simulink model "PID_HW_EKF"  (R2024a)
settings: Solver=FixedStepAuto  StartTime=0.0  StopTime=inf  FixedStep=0.001  RelTol=1e-3  EnableMultiTasking=on
undefined symbols (not defined in the file): dev, Main, MAX_CONTROL_ANGLE_RATE_ROLL, P, pwm_output0, R_p_x, Saturation_I_RP_Max, Saturation_I_RP_Min
libraries: slpidlib x5, px4Sensorslib x2, px4lib x1
settings Model: SimulationMode=external  ExtModeTrigDuration=10  Creator=ArriGE66  LastModifiedBy=sebas
settings SolverCC: PositivePriorityOrder=on
settings OptimizationCC: EnhancedBackFolding=on  PassReuseOutputArgsAs=Individual arguments  ZeroExternalMemoryAtStartup=off  ZeroInternalMemoryAtStartup=off  MaxStackSize=64  OptimizeBlockOrder=speed  DifferentSizesBufferReuse=on  EfficientTunableParamExpr=on
settings DebuggingCC: ParameterTunabilityLossMsg=error
settings HardwareCC: ProdBitPerPointer=32  ProdBitPerSizeT=32  ProdBitPerPtrDiffT=32  ProdLargestAtomicInteger=Long  ProdLargestAtomicFloat=Double  ProdWordSize=32  ProdLongLongMode=on  ProdHWDeviceType=ARM Compatible->ARM Cortex
settings SFSimCC: MATLABDynamicMemAlloc=off  SimTargetLang=C++
settings RTWCC: Description=Embedded Coder  SystemTargetFile=ert.tlc  HardwareBoard=PX4 Cube Orange  TemplateMakefile=ert_default_tmf  Toolchain=GNU Tools for PX4 Autopilots  TargetLang=C++  GPUComputeCapability=3.5
settings CodeAppCC: ForceParamTrailComments=on  IgnoreCustomStorageClasses=off  OperatorAnnotations=on  SimulinkDataObjDesc=on  SFDataObjDesc=on  InsertBlockDesc=on
settings ERTTargetCC: ExtMode=on  ExtModeTransport=3  ExtModeStaticAlloc=on  ExtModeStaticAllocSize=1024  ExtModeMexFile=ext_xcp  ExtModeMexArgs=1 COM10 3000000  ExtModeIntrfLevel=Level2 - Open

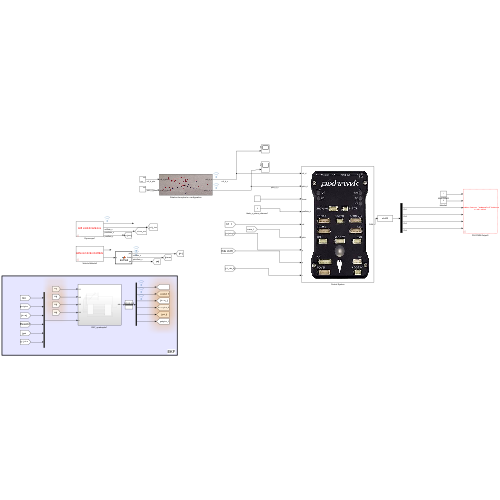
[thumbnail: Simulink's stored preview of the top-level diagram]
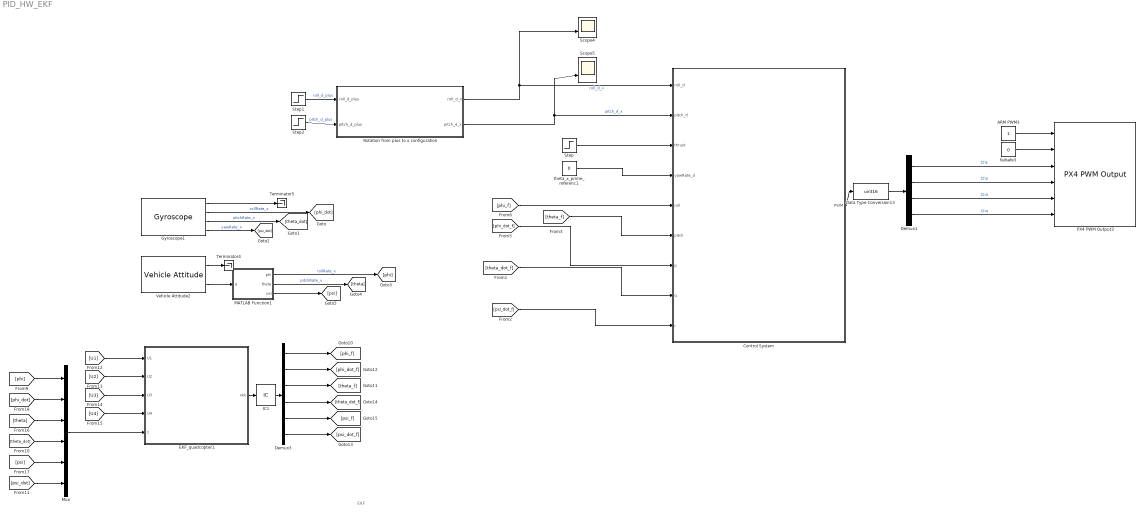
== system PID_HW_EKF ==
  note: EKF
  ARM PWM3 : Constant  OutDataTypeStr=boolean  SampleTime=0.002
  Control System : Subsystem
      mask Display: image('icon\pixhawk.png');
  Data Type Conversion13 : DataTypeConversion  OutDataTypeStr=uint16  SaturateOnIntegerOverflow=off  RndMeth=Floor
  Demux1 : Demux
  Demux3 : Demux  Outputs=6
  EKF_quadcopter1 : Subsystem
  Gyroscope1 : px4Sensorslib/Gyroscope  uorbTimeStamp=off  BlockingMode=off  BlockTimeout=1e-3  sampleTime=0.002
  IC1 : InitialCondition  Value=[0;0;0;0;0;0]
  MATLAB Function1 : MATLAB Function  TreatAsAtomicUnit=on
  Mux : Mux  Inputs=6
  PX4 PWM Output3 : px4lib/PX4 PWM Output  pwmDevice=Main (/dev/pwm_output0)  pwmChannel1_=on  pwmChannel2_=on  pwmChannel3_=on  pwmChannel4_=on  pwmChannel5_=off  pwmChannel6_=off  pwmChannel7_=off  pwmChannel8_=off  forceTerminateFailsafe=off  outputErrorStatus=off
  Rotation from plus to x configuration : Subsystem
      mask Display: image('rotation_matrix.jpg');
  Scope4 : Scope  NumInputPorts=2
  Scope5 : Scope  NumInputPorts=2
  Step : Step  After=0.6085  SampleTime=0.002
  Step1 : Step  Time=0  After=0  SampleTime=0.002
  Step2 : Step  Time=2  After=0  SampleTime=0.002
  Terminator4 : Terminator
  Terminator5 : Terminator
  Vehicle Attitude2 : px4Sensorslib/Vehicle Attitude  rollRate=off  pitchRate=off  yawRate=off  quaternion=on  uorbTimeStamp=off  BlockingMode=off  BlockTimeout=0.001  sampleTime=0.002
  failsafe3 : Constant  Value=0  OutDataTypeStr=boolean  SampleTime=0.002
  theta_x_prime_referenc1 : Constant  Value=0  SampleTime=0.002
  wires:
  Control System/1(PWM) -> Data Type Conversion13/1
  Data Type Conversion13/1 -> Demux1/1
  Demux1/1 -> PX4 PWM Output3/3  "Ch1"
  Demux1/2 -> PX4 PWM Output3/4  "Ch2"
  ARM PWM3/1 -> PX4 PWM Output3/1
  failsafe3/1 -> PX4 PWM Output3/2
  Step/1 -> Control System/3(thrust)
  theta_x_prime_referenc1/1 -> Control System/4(yawRate_d)
  Demux1/3 -> PX4 PWM Output3/5  "Ch3"
  Demux1/4 -> PX4 PWM Output3/6  "Ch4"
  Rotation from plus to x configuration/2(pitch_d_x) -> Control System/2(pitch_d), Scope5/2  "pitch_d_x"
  Rotation from plus to x configuration/1(roll_d_x) -> Control System/1(roll_d), Scope4/2  "roll_d_x"
  Step1/1 -> Rotation from plus to x configuration/1(roll_d_plus)  "roll_d_plus"
  Step2/1 -> Rotation from plus to x configuration/2(pitch_d_plus)  "pitch_d_plus"
  MATLAB Function1/2(theta) -> [theta]  "pitchRate_x"
  MATLAB Function1/1(phi) -> [phi]  "rollRate_x"
  Gyroscope1/1 -> Terminator5/1
  Vehicle Attitude2/2 -> MATLAB Function1/1(q)
  Vehicle Attitude2/1 -> Terminator4/1
  Gyroscope1/3 -> [theta_dot]  "pitchRate_x"
  Gyroscope1/2 -> [phi_dot]  "rollRate_x"
  Gyroscope1/4 -> [psi_dot]  "yawRate_x"
  MATLAB Function1/3(psi) -> [psi]
  [U1] -> EKF_quadcopter1/1(U1)
  Mux/1 -> EKF_quadcopter1/5(z)
  [phi] -> Mux/1
  [U3] -> EKF_quadcopter1/3(U3)
  [psi_dot] -> Mux/6
  [U2] -> EKF_quadcopter1/2(U2)
  [psi] -> Mux/5
  Demux3/5 -> [psi_f]
  [theta] -> Mux/3
  [theta_dot] -> Mux/4
  Demux3/2 -> [phi_dot_f]
  Demux3/1 -> [phi_f]
  Demux3/6 -> [psi_dot_f]
  EKF_quadcopter1/1(xkk) -> IC1/1
  Demux3/3 -> [theta_f]
  [phi_dot] -> Mux/2
  Demux3/4 -> [theta_dot_f]
  IC1/1 -> Demux3/1
  [U4] -> EKF_quadcopter1/4(U4)
  [theta_dot_f] -> Control System/8(q)
  [theta_f] -> Control System/6(pitch)
  [psi_dot_f] -> Control System/9(r)
  [phi_f] -> Control System/5(roll)
  [phi_dot_f] -> Control System/7(p)

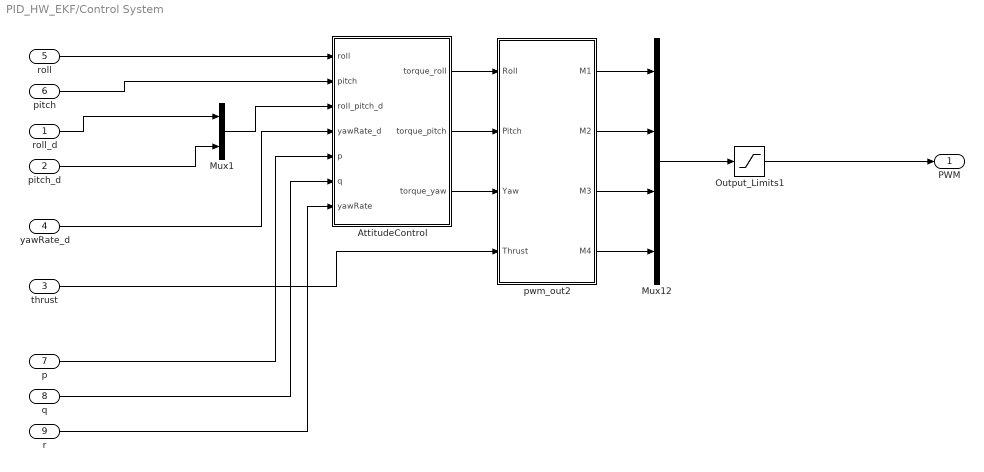
== system PID_HW_EKF/Control System ==
  roll_d : Inport  PortDimensions=1
  pitch_d : Inport  Port=2  PortDimensions=1
  thrust : Inport  Port=3  PortDimensions=1
  yawRate_d : Inport  Port=4  PortDimensions=1
  roll : Inport  Port=5  PortDimensions=1
  pitch : Inport  Port=6  PortDimensions=1
  p : Inport  Port=7  PortDimensions=1
  q : Inport  Port=8  PortDimensions=1
  r : Inport  Port=9  PortDimensions=1
  AttitudeControl : Subsystem
  Mux1 : Mux  Inputs=2
  Mux12 : Mux
  Output_Limits1 : Saturate  UpperLimit=2000  LowerLimit=1000  LinearizeAsGain=off
  pwm_out2 : MATLAB Function  SystemSampleTime=0.004
  PWM : Outport  VectorParamsAs1DForOutWhenUnconnected=off
  wires:
  thrust/1 -> pwm_out2/4(Thrust)
  Mux12/1 -> Output_Limits1/1
  AttitudeControl/2(torque_pitch) -> pwm_out2/2(Pitch)
  AttitudeControl/1(torque_roll) -> pwm_out2/1(Roll)
  pwm_out2/1(M1) -> Mux12/1
  pwm_out2/3(M3) -> Mux12/3
  pwm_out2/2(M2) -> Mux12/2
  r/1 -> AttitudeControl/7(yawRate)
  AttitudeControl/3(torque_yaw) -> pwm_out2/3(Yaw)
  Mux1/1 -> AttitudeControl/3(roll_pitch_d)
  q/1 -> AttitudeControl/6(q)
  yawRate_d/1 -> AttitudeControl/4(yawRate_d)
  p/1 -> AttitudeControl/5(p)
  pwm_out2/4(M4) -> Mux12/4
  pitch/1 -> AttitudeControl/2(pitch)
  roll/1 -> AttitudeControl/1(roll)
  Output_Limits1/1 -> PWM/1
  roll_d/1 -> Mux1/1
  pitch_d/1 -> Mux1/2

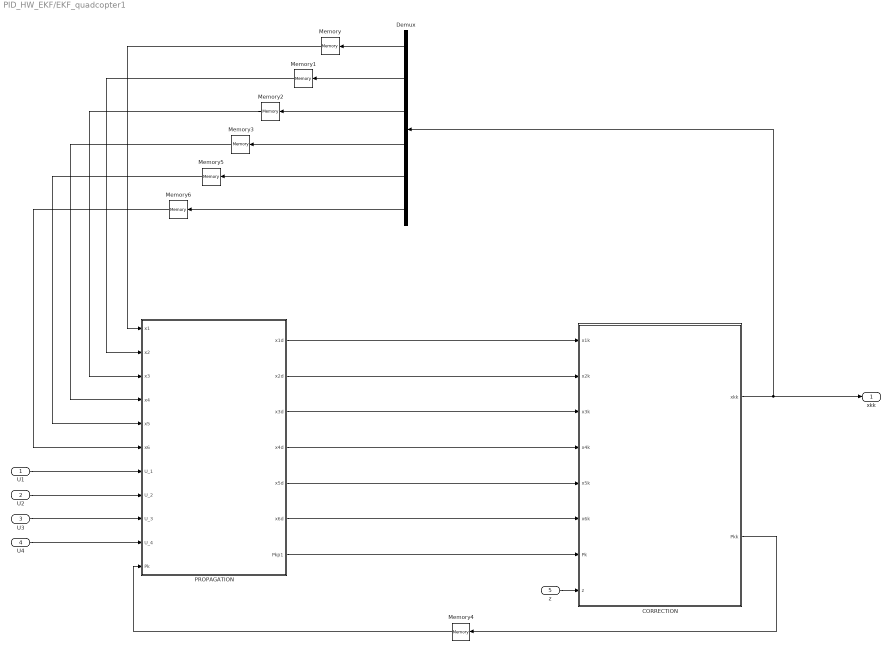
== system PID_HW_EKF/EKF_quadcopter1 ==
  U1 : Inport
  U2 : Inport  Port=2
  U3 : Inport  Port=3
  U4 : Inport  Port=4
  z : Inport  Port=5
  CORRECTION : MATLAB Function  TreatAsAtomicUnit=on
  Demux : Demux  Outputs=6
  Memory{,1..3,5..6} (6 alike) : Memory
  Memory4 : Memory  InitialCondition=P
  PROPAGATION : MATLAB Function  TreatAsAtomicUnit=on
  xkk : Outport
  wires:
  PROPAGATION/1(x1d) -> CORRECTION/1(x1k)
  PROPAGATION/2(x2d) -> CORRECTION/2(x2k)
  PROPAGATION/3(x3d) -> CORRECTION/3(x3k)
  PROPAGATION/4(x4d) -> CORRECTION/4(x4k)
  Memory4/1 -> PROPAGATION/11(Pk)
  U1/1 -> PROPAGATION/7(U_1)
  U2/1 -> PROPAGATION/8(U_2)
  U3/1 -> PROPAGATION/9(U_3)
  U4/1 -> PROPAGATION/10(U_4)
  PROPAGATION/7(Pkp1) -> CORRECTION/7(Pk)
  CORRECTION/2(Pkk) -> Memory4/1
  z/1 -> CORRECTION/8(z)
  Demux/1 -> Memory/1
  Demux/2 -> Memory1/1
  Demux/3 -> Memory2/1
  Demux/4 -> Memory3/1
  CORRECTION/1(xkk) -> Demux/1, xkk/1
  Memory/1 -> PROPAGATION/1(x1)
  Memory1/1 -> PROPAGATION/2(x2)
  Memory2/1 -> PROPAGATION/3(x3)
  Memory3/1 -> PROPAGATION/4(x4)
  PROPAGATION/6(x6d) -> CORRECTION/6(x6k)
  PROPAGATION/5(x5d) -> CORRECTION/5(x5k)
  Demux/5 -> Memory5/1
  Memory5/1 -> PROPAGATION/5(x5)
  Demux/6 -> Memory6/1
  Memory6/1 -> PROPAGATION/6(x6)

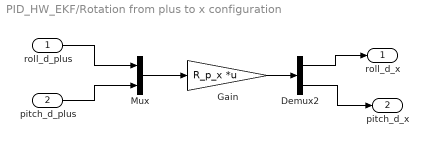
== system PID_HW_EKF/Rotation from plus to x configuration ==
  roll_d_plus : Inport
  pitch_d_plus : Inport  Port=2
  Demux2 : Demux  Outputs=2
  Gain : Gain  Gain=R_p_x  Multiplication=Matrix(K*u) (u vector)
  Mux : Mux  Inputs=2
  roll_d_x : Outport
  pitch_d_x : Outport  Port=2
  wires:
  roll_d_plus/1 -> Mux/1
  Mux/1 -> Gain/1
  Demux2/1 -> roll_d_x/1
  Gain/1 -> Demux2/1
  pitch_d_plus/1 -> Mux/2
  Demux2/2 -> pitch_d_x/1

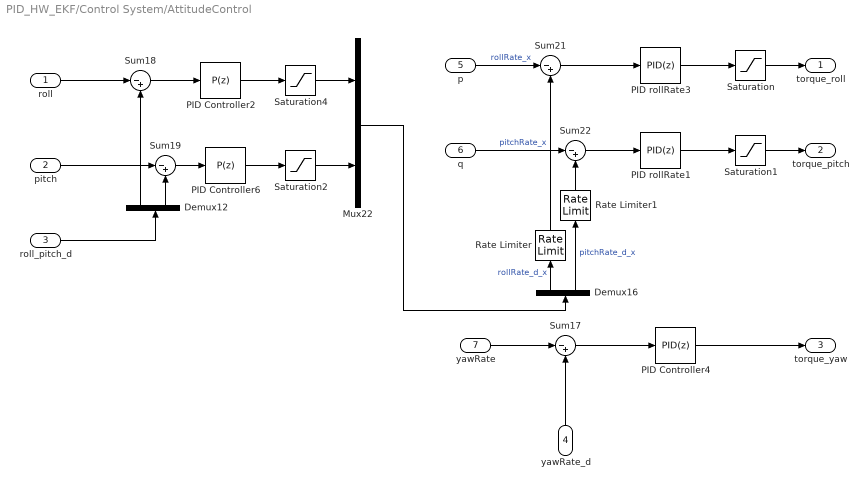
== system PID_HW_EKF/Control System/AttitudeControl ==
  roll : Inport
  pitch : Inport  Port=2
  roll_pitch_d : Inport  Port=3
  yawRate_d : Inport  Port=4
  p : Inport  Port=5
  q : Inport  Port=6
  yawRate : Inport  Port=7
  Demux12 : Demux  Outputs=2
  Demux16 : Demux  Outputs=2
  Mux22 : Mux  Inputs=2
  PID Controller2 : slpidlib/PID Controller  Controller=P  Form=Parallel  TimeDomain=Discrete-time  UseExternalTs=off  SampleTime=-1  IntegratorMethod=Forward Euler  FilterMethod=Forward Euler  ControllerParametersSource=internal  P=2.809480033162003  I=1  UseKiTs=off  D=0  UseExternalDerivativeSource=off  N=100  UseFilter=on  TunerSelectOption=Transfer Function Based (PID Tuner App)  InitialConditionSource=internal  InitialConditionForIntegrator=0  InitialConditionForFilter=0  DifferentiatorICPrevScaledInput=0  ExternalReset=none  TrackingMode=off  Kt=1  LimitOutput=off  SatLimitsSource=internal  UpperSaturationLimit=inf  LowerSaturationLimit=-inf  LinearizeAsGain=on  AntiWindupMode=none  Kb=1  LimitIntegrator=off  UpperIntegratorSaturationLimit=inf  LowerIntegratorSaturationLimit=-inf  POutMin=[]  POutMax=[]  IOutMin=[]  IOutMax=[]  DOutMin=[]  DOutMax=[]  NOutMin=[]  NOutMax=[]  SumOutMin=[]  SumOutMax=[]  SaturationOutMin=[]  SaturationOutMax=[]  PParamMin=[]  PParamMax=[]  IParamMin=[]  IParamMax=[]  DParamMin=[]  DParamMax=[]  NParamMin=[]  NParamMax=[]  KbParamMin=[]  KbParamMax=[]  KtParamMin=[]  KtParamMax=[]  KbOutMin=[]  KbOutMax=[]  KtOutMin=[]  KtOutMax=[]  IntegratorOutMin=[]  IntegratorOutMax=[]  FilterOutMin=[]  FilterOutMax=[]  SumI1OutMin=[]  SumI1OutMax=[]  SumI2OutMin=[]  SumI2OutMax=[]  SumI3OutMin=[]  SumI3OutMax=[]  SumI4OutMin=[]  SumI4OutMax=[]  SumDOutMin=[]  SumDOutMax=[]  DifferentiatorOutMin=[]  DifferentiatorOutMax=[]  FilterDiffOutCoefMin=[]  FilterDiffOutCoefMax=[]  ReciprocalOutMin=[]  ReciprocalOutMax=[]  SumDenOutMin=[]  SumDenOutMax=[]  SumNumOutMin=[]  SumNumOutMax=[]  DivideOutMin=[]  DivideOutMax=[]  UdiffTsProdOutMin=[]  UdiffTsProdOutMax=[]  NTsProdOutMin=[]  NTsProdOutMax=[]  UintegralTsProdOutMin=[]  UintegralTsProdOutMax=[]  UngainTsProdOutMin=[]  UngainTsProdOutMax=[]  ClampingZeroOutDataTypeStr=Inherit: Inherit via back propagation  ClampingZeroOutMin=[]  ClampingZeroOutMax=[]  FilterDenConstantOutDataTypeStr=Inherit: Inherit via back propagation  FilterDenConstantOutMin=[]  FilterDenConstantOutMax=[]  PCopyOutDataTypeStr=Inherit: Inherit via back propagation  PCopyOutMin=[]  PCopyOutMax=[]  NCopyOutDataTypeStr=Inherit: Inherit via back propagation  NCopyOutMin=[]  NCopyOutMax=[]  IntegratorContinuousStateAttributes=''  IntegratorStateMustResolveToSignalObject=off  IntegratorRTWStateStorageClass=Auto  FilterContinuousStateAttributes=''  FilterStateMustResolveToSignalObject=off  FilterRTWStateStorageClass=Auto  ParallelPVariant=InternalParameters  IdealPVariant=Disabled  IVariant=Disabled  DVariant=Disabled  IntegratorVariant=Disabled  SatVariant=Disabled  AWVariant=Disabled  PCopyVariant=Disabled  TRVariant=Disabled  FdbkBlocksVariant=Forward  IdealPFdbkVariant=Disabled  SatFdbkVariant=Disabled  DerivativeFilterVariant=Disabled  NVariant=Disabled  NCopyVariant=Disabled_SignalSpec  FilterICVariant=Disabled  IntegratorICVariant=Disabled  ExternalResetVariant=Disabled  TRSumVariant=Passthrough  SumFdbkVariant=Disabled  SumVariant=Passthrough_P  TsampFilterVariant=InternalTs  TsampNgainVariant=Passthrough  TsampIntegralVariant=Disabled_SignalSpec  ExternalSaturationOutDataTypeStr=Inherit: Same as second input  DerivativeSourceVariant=Disabled
  PID Controller4 : slpidlib/PID Controller  Controller=PID  Form=Parallel  TimeDomain=Discrete-time  UseExternalTs=off  SampleTime=-1  IntegratorMethod=Forward Euler  FilterMethod=Forward Euler  ControllerParametersSource=internal  P=7.29164976020127  I=128.977906817925  UseKiTs=off  D=0.0102787963324955  UseExternalDerivativeSource=off  N=308.658502253511  UseFilter=on  TunerSelectOption=Transfer Function Based (PID Tuner App)  InitialConditionSource=internal  InitialConditionForIntegrator=0  InitialConditionForFilter=0  DifferentiatorICPrevScaledInput=0  ExternalReset=none  TrackingMode=off  Kt=1  LimitOutput=off  SatLimitsSource=internal  UpperSaturationLimit=Saturation_I_RP_Max  LowerSaturationLimit=Saturation_I_RP_Min  LinearizeAsGain=on  AntiWindupMode=none  Kb=1  LimitIntegrator=off  UpperIntegratorSaturationLimit=inf  LowerIntegratorSaturationLimit=-inf  POutMin=[]  POutMax=[]  IOutMin=[]  IOutMax=[]  DOutMin=[]  DOutMax=[]  NOutMin=[]  NOutMax=[]  SumOutMin=[]  SumOutMax=[]  SaturationOutMin=[]  SaturationOutMax=[]  PParamMin=[]  PParamMax=[]  IParamMin=[]  IParamMax=[]  DParamMin=[]  DParamMax=[]  NParamMin=[]  NParamMax=[]  KbParamMin=[]  KbParamMax=[]  KtParamMin=[]  KtParamMax=[]  KbOutMin=[]  KbOutMax=[]  KtOutMin=[]  KtOutMax=[]  IntegratorOutMin=[]  IntegratorOutMax=[]  FilterOutMin=[]  FilterOutMax=[]  SumI1OutMin=[]  SumI1OutMax=[]  SumI2OutMin=[]  SumI2OutMax=[]  SumI3OutMin=[]  SumI3OutMax=[]  SumI4OutMin=[]  SumI4OutMax=[]  SumDOutMin=[]  SumDOutMax=[]  DifferentiatorOutMin=[]  DifferentiatorOutMax=[]  FilterDiffOutCoefMin=[]  FilterDiffOutCoefMax=[]  ReciprocalOutMin=[]  ReciprocalOutMax=[]  SumDenOutMin=[]  SumDenOutMax=[]  SumNumOutMin=[]  SumNumOutMax=[]  DivideOutMin=[]  DivideOutMax=[]  UdiffTsProdOutMin=[]  UdiffTsProdOutMax=[]  NTsProdOutMin=[]  NTsProdOutMax=[]  UintegralTsProdOutMin=[]  UintegralTsProdOutMax=[]  UngainTsProdOutMin=[]  UngainTsProdOutMax=[]  ClampingZeroOutDataTypeStr=Inherit: Inherit via back propagation  ClampingZeroOutMin=[]  ClampingZeroOutMax=[]  FilterDenConstantOutDataTypeStr=Inherit: Inherit via back propagation  FilterDenConstantOutMin=[]  FilterDenConstantOutMax=[]  PCopyOutDataTypeStr=Inherit: Inherit via back propagation  PCopyOutMin=[]  PCopyOutMax=[]  NCopyOutDataTypeStr=Inherit: Inherit via back propagation  NCopyOutMin=[]  NCopyOutMax=[]  IntegratorContinuousStateAttributes=''  IntegratorStateMustResolveToSignalObject=off  IntegratorRTWStateStorageClass=Auto  FilterContinuousStateAttributes=''  FilterStateMustResolveToSignalObject=off  FilterRTWStateStorageClass=Auto  ParallelPVariant=InternalParameters  IdealPVariant=Disabled  IVariant=InternalParameters  DVariant=InternalParameters  IntegratorVariant=Discrete  SatVariant=Disabled  AWVariant=Passthrough  PCopyVariant=Disabled  TRVariant=Disabled  FdbkBlocksVariant=Forward  IdealPFdbkVariant=Disabled  SatFdbkVariant=Disabled  DerivativeFilterVariant=ForwardEulerFilter  NVariant=InternalParameters  NCopyVariant=Disabled  FilterICVariant=InternalICsFilter  IntegratorICVariant=InternalICs  ExternalResetVariant=Disabled  TRSumVariant=Passthrough  SumFdbkVariant=Disabled  SumVariant=Sum_PID  TsampFilterVariant=InternalTs  TsampNgainVariant=Passthrough  TsampIntegralVariant=Disabled_SignalSpec  ExternalSaturationOutDataTypeStr=Inherit: Same as second input  DerivativeSourceVariant=ErrorSignal
  PID Controller6 : slpidlib/PID Controller  Controller=P  Form=Parallel  TimeDomain=Discrete-time  UseExternalTs=off  SampleTime=-1  IntegratorMethod=Forward Euler  FilterMethod=Forward Euler  ControllerParametersSource=internal  P=2.809480033162003  I=1  UseKiTs=off  D=0  UseExternalDerivativeSource=off  N=100  UseFilter=on  TunerSelectOption=Transfer Function Based (PID Tuner App)  InitialConditionSource=internal  InitialConditionForIntegrator=0  InitialConditionForFilter=0  DifferentiatorICPrevScaledInput=0  ExternalReset=none  TrackingMode=off  Kt=1  LimitOutput=off  SatLimitsSource=internal  UpperSaturationLimit=inf  LowerSaturationLimit=-inf  LinearizeAsGain=on  AntiWindupMode=none  Kb=1  LimitIntegrator=off  UpperIntegratorSaturationLimit=inf  LowerIntegratorSaturationLimit=-inf  POutMin=[]  POutMax=[]  IOutMin=[]  IOutMax=[]  DOutMin=[]  DOutMax=[]  NOutMin=[]  NOutMax=[]  SumOutMin=[]  SumOutMax=[]  SaturationOutMin=[]  SaturationOutMax=[]  PParamMin=[]  PParamMax=[]  IParamMin=[]  IParamMax=[]  DParamMin=[]  DParamMax=[]  NParamMin=[]  NParamMax=[]  KbParamMin=[]  KbParamMax=[]  KtParamMin=[]  KtParamMax=[]  KbOutMin=[]  KbOutMax=[]  KtOutMin=[]  KtOutMax=[]  IntegratorOutMin=[]  IntegratorOutMax=[]  FilterOutMin=[]  FilterOutMax=[]  SumI1OutMin=[]  SumI1OutMax=[]  SumI2OutMin=[]  SumI2OutMax=[]  SumI3OutMin=[]  SumI3OutMax=[]  SumI4OutMin=[]  SumI4OutMax=[]  SumDOutMin=[]  SumDOutMax=[]  DifferentiatorOutMin=[]  DifferentiatorOutMax=[]  FilterDiffOutCoefMin=[]  FilterDiffOutCoefMax=[]  ReciprocalOutMin=[]  ReciprocalOutMax=[]  SumDenOutMin=[]  SumDenOutMax=[]  SumNumOutMin=[]  SumNumOutMax=[]  DivideOutMin=[]  DivideOutMax=[]  UdiffTsProdOutMin=[]  UdiffTsProdOutMax=[]  NTsProdOutMin=[]  NTsProdOutMax=[]  UintegralTsProdOutMin=[]  UintegralTsProdOutMax=[]  UngainTsProdOutMin=[]  UngainTsProdOutMax=[]  ClampingZeroOutDataTypeStr=Inherit: Inherit via back propagation  ClampingZeroOutMin=[]  ClampingZeroOutMax=[]  FilterDenConstantOutDataTypeStr=Inherit: Inherit via back propagation  FilterDenConstantOutMin=[]  FilterDenConstantOutMax=[]  PCopyOutDataTypeStr=Inherit: Inherit via back propagation  PCopyOutMin=[]  PCopyOutMax=[]  NCopyOutDataTypeStr=Inherit: Inherit via back propagation  NCopyOutMin=[]  NCopyOutMax=[]  IntegratorContinuousStateAttributes=''  IntegratorStateMustResolveToSignalObject=off  IntegratorRTWStateStorageClass=Auto  FilterContinuousStateAttributes=''  FilterStateMustResolveToSignalObject=off  FilterRTWStateStorageClass=Auto  ParallelPVariant=InternalParameters  IdealPVariant=Disabled  IVariant=Disabled  DVariant=Disabled  IntegratorVariant=Disabled  SatVariant=Disabled  AWVariant=Disabled  PCopyVariant=Disabled  TRVariant=Disabled  FdbkBlocksVariant=Forward  IdealPFdbkVariant=Disabled  SatFdbkVariant=Disabled  DerivativeFilterVariant=Disabled  NVariant=Disabled  NCopyVariant=Disabled_SignalSpec  FilterICVariant=Disabled  IntegratorICVariant=Disabled  ExternalResetVariant=Disabled  TRSumVariant=Passthrough  SumFdbkVariant=Disabled  SumVariant=Passthrough_P  TsampFilterVariant=InternalTs  TsampNgainVariant=Passthrough  TsampIntegralVariant=Disabled_SignalSpec  ExternalSaturationOutDataTypeStr=Inherit: Same as second input  DerivativeSourceVariant=Disabled
  PID rollRate1 : slpidlib/PID Controller  Controller=PID  Form=Parallel  TimeDomain=Discrete-time  UseExternalTs=off  SampleTime=-1  IntegratorMethod=Forward Euler  FilterMethod=Forward Euler  ControllerParametersSource=internal  P=7.82928757295584  I=30.614354689847  UseKiTs=off  D=-0.0391699970557117  UseExternalDerivativeSource=off  N=24.5460626191563  UseFilter=on  TunerSelectOption=Transfer Function Based (PID Tuner App)  InitialConditionSource=internal  InitialConditionForIntegrator=0  InitialConditionForFilter=0  DifferentiatorICPrevScaledInput=0  ExternalReset=none  TrackingMode=off  Kt=1  LimitOutput=off  SatLimitsSource=internal  UpperSaturationLimit=Saturation_I_RP_Max  LowerSaturationLimit=Saturation_I_RP_Min  LinearizeAsGain=on  AntiWindupMode=none  Kb=1  LimitIntegrator=off  UpperIntegratorSaturationLimit=inf  LowerIntegratorSaturationLimit=-inf  POutMin=[]  POutMax=[]  IOutMin=[]  IOutMax=[]  DOutMin=[]  DOutMax=[]  NOutMin=[]  NOutMax=[]  SumOutMin=[]  SumOutMax=[]  SaturationOutMin=[]  SaturationOutMax=[]  PParamMin=[]  PParamMax=[]  IParamMin=[]  IParamMax=[]  DParamMin=[]  DParamMax=[]  NParamMin=[]  NParamMax=[]  KbParamMin=[]  KbParamMax=[]  KtParamMin=[]  KtParamMax=[]  KbOutMin=[]  KbOutMax=[]  KtOutMin=[]  KtOutMax=[]  IntegratorOutMin=[]  IntegratorOutMax=[]  FilterOutMin=[]  FilterOutMax=[]  SumI1OutMin=[]  SumI1OutMax=[]  SumI2OutMin=[]  SumI2OutMax=[]  SumI3OutMin=[]  SumI3OutMax=[]  SumI4OutMin=[]  SumI4OutMax=[]  SumDOutMin=[]  SumDOutMax=[]  DifferentiatorOutMin=[]  DifferentiatorOutMax=[]  FilterDiffOutCoefMin=[]  FilterDiffOutCoefMax=[]  ReciprocalOutMin=[]  ReciprocalOutMax=[]  SumDenOutMin=[]  SumDenOutMax=[]  SumNumOutMin=[]  SumNumOutMax=[]  DivideOutMin=[]  DivideOutMax=[]  UdiffTsProdOutMin=[]  UdiffTsProdOutMax=[]  NTsProdOutMin=[]  NTsProdOutMax=[]  UintegralTsProdOutMin=[]  UintegralTsProdOutMax=[]  UngainTsProdOutMin=[]  UngainTsProdOutMax=[]  ClampingZeroOutDataTypeStr=Inherit: Inherit via back propagation  ClampingZeroOutMin=[]  ClampingZeroOutMax=[]  FilterDenConstantOutDataTypeStr=Inherit: Inherit via back propagation  FilterDenConstantOutMin=[]  FilterDenConstantOutMax=[]  PCopyOutDataTypeStr=Inherit: Inherit via back propagation  PCopyOutMin=[]  PCopyOutMax=[]  NCopyOutDataTypeStr=Inherit: Inherit via back propagation  NCopyOutMin=[]  NCopyOutMax=[]  IntegratorContinuousStateAttributes=''  IntegratorStateMustResolveToSignalObject=off  IntegratorRTWStateStorageClass=Auto  FilterContinuousStateAttributes=''  FilterStateMustResolveToSignalObject=off  FilterRTWStateStorageClass=Auto  ParallelPVariant=InternalParameters  IdealPVariant=Disabled  IVariant=InternalParameters  DVariant=InternalParameters  IntegratorVariant=Discrete  SatVariant=Disabled  AWVariant=Passthrough  PCopyVariant=Disabled  TRVariant=Disabled  FdbkBlocksVariant=Forward  IdealPFdbkVariant=Disabled  SatFdbkVariant=Disabled  DerivativeFilterVariant=ForwardEulerFilter  NVariant=InternalParameters  NCopyVariant=Disabled  FilterICVariant=InternalICsFilter  IntegratorICVariant=InternalICs  ExternalResetVariant=Disabled  TRSumVariant=Passthrough  SumFdbkVariant=Disabled  SumVariant=Sum_PID  TsampFilterVariant=InternalTs  TsampNgainVariant=Passthrough  TsampIntegralVariant=Disabled_SignalSpec  ExternalSaturationOutDataTypeStr=Inherit: Same as second input  DerivativeSourceVariant=ErrorSignal
  PID rollRate3 : slpidlib/PID Controller  Controller=PID  Form=Parallel  TimeDomain=Discrete-time  UseExternalTs=off  SampleTime=-1  IntegratorMethod=Forward Euler  FilterMethod=Forward Euler  ControllerParametersSource=internal  P=7.82928757295584  I=30.614354689847  UseKiTs=off  D=-0.0391699970557117  UseExternalDerivativeSource=off  N=24.5460626191563  UseFilter=on  TunerSelectOption=Transfer Function Based (PID Tuner App)  InitialConditionSource=internal  InitialConditionForIntegrator=0  InitialConditionForFilter=0  DifferentiatorICPrevScaledInput=0  ExternalReset=none  TrackingMode=off  Kt=1  LimitOutput=off  SatLimitsSource=internal  UpperSaturationLimit=Saturation_I_RP_Max  LowerSaturationLimit=Saturation_I_RP_Min  LinearizeAsGain=on  AntiWindupMode=none  Kb=1  LimitIntegrator=off  UpperIntegratorSaturationLimit=inf  LowerIntegratorSaturationLimit=-inf  POutMin=[]  POutMax=[]  IOutMin=[]  IOutMax=[]  DOutMin=[]  DOutMax=[]  NOutMin=[]  NOutMax=[]  SumOutMin=[]  SumOutMax=[]  SaturationOutMin=[]  SaturationOutMax=[]  PParamMin=[]  PParamMax=[]  IParamMin=[]  IParamMax=[]  DParamMin=[]  DParamMax=[]  NParamMin=[]  NParamMax=[]  KbParamMin=[]  KbParamMax=[]  KtParamMin=[]  KtParamMax=[]  KbOutMin=[]  KbOutMax=[]  KtOutMin=[]  KtOutMax=[]  IntegratorOutMin=[]  IntegratorOutMax=[]  FilterOutMin=[]  FilterOutMax=[]  SumI1OutMin=[]  SumI1OutMax=[]  SumI2OutMin=[]  SumI2OutMax=[]  SumI3OutMin=[]  SumI3OutMax=[]  SumI4OutMin=[]  SumI4OutMax=[]  SumDOutMin=[]  SumDOutMax=[]  DifferentiatorOutMin=[]  DifferentiatorOutMax=[]  FilterDiffOutCoefMin=[]  FilterDiffOutCoefMax=[]  ReciprocalOutMin=[]  ReciprocalOutMax=[]  SumDenOutMin=[]  SumDenOutMax=[]  SumNumOutMin=[]  SumNumOutMax=[]  DivideOutMin=[]  DivideOutMax=[]  UdiffTsProdOutMin=[]  UdiffTsProdOutMax=[]  NTsProdOutMin=[]  NTsProdOutMax=[]  UintegralTsProdOutMin=[]  UintegralTsProdOutMax=[]  UngainTsProdOutMin=[]  UngainTsProdOutMax=[]  ClampingZeroOutDataTypeStr=Inherit: Inherit via back propagation  ClampingZeroOutMin=[]  ClampingZeroOutMax=[]  FilterDenConstantOutDataTypeStr=Inherit: Inherit via back propagation  FilterDenConstantOutMin=[]  FilterDenConstantOutMax=[]  PCopyOutDataTypeStr=Inherit: Inherit via back propagation  PCopyOutMin=[]  PCopyOutMax=[]  NCopyOutDataTypeStr=Inherit: Inherit via back propagation  NCopyOutMin=[]  NCopyOutMax=[]  IntegratorContinuousStateAttributes=''  IntegratorStateMustResolveToSignalObject=off  IntegratorRTWStateStorageClass=Auto  FilterContinuousStateAttributes=''  FilterStateMustResolveToSignalObject=off  FilterRTWStateStorageClass=Auto  ParallelPVariant=InternalParameters  IdealPVariant=Disabled  IVariant=InternalParameters  DVariant=InternalParameters  IntegratorVariant=Discrete  SatVariant=Disabled  AWVariant=Passthrough  PCopyVariant=Disabled  TRVariant=Disabled  FdbkBlocksVariant=Forward  IdealPFdbkVariant=Disabled  SatFdbkVariant=Disabled  DerivativeFilterVariant=ForwardEulerFilter  NVariant=InternalParameters  NCopyVariant=Disabled  FilterICVariant=InternalICsFilter  IntegratorICVariant=InternalICs  ExternalResetVariant=Disabled  TRSumVariant=Passthrough  SumFdbkVariant=Disabled  SumVariant=Sum_PID  TsampFilterVariant=InternalTs  TsampNgainVariant=Passthrough  TsampIntegralVariant=Disabled_SignalSpec  ExternalSaturationOutDataTypeStr=Inherit: Same as second input  DerivativeSourceVariant=ErrorSignal
  Rate Limiter : RateLimiter  SampleTimeMode=inherited
  Rate Limiter1 : RateLimiter  SampleTimeMode=inherited
  Saturation : Saturate  UpperLimit=1  LowerLimit=-1
  Saturation1 : Saturate  UpperLimit=1  LowerLimit=-1
  Saturation2 : Saturate  UpperLimit=MAX_CONTROL_ANGLE_RATE_ROLL  LowerLimit=-MAX_CONTROL_ANGLE_RATE_ROLL
  Saturation4 : Saturate  UpperLimit=MAX_CONTROL_ANGLE_RATE_ROLL  LowerLimit=-MAX_CONTROL_ANGLE_RATE_ROLL
  Sum{17..19,21..22} (5 alike) : Sum  Inputs=|-+
  torque_roll : Outport  VectorParamsAs1DForOutWhenUnconnected=off
  torque_pitch : Outport  Port=2  VectorParamsAs1DForOutWhenUnconnected=off
  torque_yaw : Outport  Port=3  VectorParamsAs1DForOutWhenUnconnected=off
  wires:
  yawRate/1 -> Sum17/1
  Sum19/1 -> PID Controller6/1
  roll/1 -> Sum18/1
  pitch/1 -> Sum19/1
  Sum18/1 -> PID Controller2/1
  Sum22/1 -> PID rollRate1/1
  p/1 -> Sum21/1  "rollRate_x"
  q/1 -> Sum22/1  "pitchRate_x"
  Sum21/1 -> PID rollRate3/1
  roll_pitch_d/1 -> Demux12/1
  Mux22/1 -> Demux16/1
  PID Controller4/1 -> torque_yaw/1
  Demux16/1 -> Rate Limiter/1  "rollRate_d_x"
  Demux12/2 -> Sum19/2
  Demux12/1 -> Sum18/2
  Demux16/2 -> Rate Limiter1/1  "pitchRate_d_x"
  Sum17/1 -> PID Controller4/1
  yawRate_d/1 -> Sum17/2
  Rate Limiter/1 -> Sum21/2
  Rate Limiter1/1 -> Sum22/2
  PID rollRate3/1 -> Saturation/1
  Saturation/1 -> torque_roll/1
  Saturation1/1 -> torque_pitch/1
  PID Controller2/1 -> Saturation4/1
  Saturation4/1 -> Mux22/1
  PID Controller6/1 -> Saturation2/1
  Saturation2/1 -> Mux22/2
  PID rollRate1/1 -> Saturation1/1

== matlab function PID_HW_EKF/Control System/pwm_out2 ==
  data: Roll input; M1 output; Pitch input; Yaw input; Thrust input; M2 output; M3 output; M4 output
function [M1, M2, M3, M4] = motor_mixer(Roll, Pitch, Yaw, Thrust)
%Function description:
%  Control allocation. The quadrotor type is X-configuration,
%  and the airframe is as follows:
%3↓   1↑
 %  \ /
 %  / \
 %2↑   4↓
%Input：
%  Roll, Pitch, Yaw: attitude controller output.
%  Thrust

idle_PWM = 1000;
scale = 1000;


M1 = (Thrust - Roll + Pitch + Yaw) * scale + idle_PWM;
M2 = (Thrust + Roll - Pitch + Yaw) * scale + idle_PWM;
M3 = (Thrust + Roll + Pitch - Yaw) * scale + idle_PWM;
M4 = (Thrust - Roll - Pitch - Yaw) * scale + idle_PWM;

== matlab function PID_HW_EKF/MATLAB Function1 ==
  data: q input; phi output; theta output; psi output
function [phi,theta,psi] = quat2eul(q)
% Conversion from Quaternion to Euler angles based on the PX4 Firmware
% v1.6.5 release.
% 
% Quaternion -> DCM -> Euler Angles
% INPUT:
%   q: Quaternion vector of the format: (a + bi + cj + dk)
% OUTPUT:
%   [phi,theta,psi]: Euler angles in radians.
% 
 
    a = q(1);
    b = q(2);
    c = q(3);
    d = q(4);

    aSq = a*a;
    bSq = b*b;
    cSq = c*c;
    dSq = d*d;

    d_pi2 = pi/2;

    % quaternion_to_dcm
    dcm00 = aSq + bSq - cSq - dSq;
    % dcm01 = 2*(b*c - a*d);
    dcm02 = 2*(a*c + b*d);
    dcm10 = 2*(b*c + a*d);
    % dcm11 = aSq - bSq + cSq - dSq;
    dcm12 = 2*(c*d - a*b);
    dcm20 = 2*(b*d - a*c);
    dcm21 = 2*(a*b + c*d);
    dcm22 = aSq - bSq - cSq + dSq;

    % dcm_to_euler
    theta = asin(-dcm20);
    if abs(theta - d_pi2) < 1.0e-3
        phi = single(0.0);
        psi = atan2(dcm12, dcm02);
    elseif abs(theta + d_pi2) < 1.0e-3
        phi = single(0.0);
        psi = atan2(-dcm12, -dcm02);
    else
        phi = atan2(dcm21, dcm22);
        psi = atan2(dcm10, dcm00);
    end

end

== matlab function PID_HW_EKF/EKF_quadcopter1/CORRECTION ==
  data: x1k input; xkk output; Pkk output; x2k input; x3k input; x4k input; x5k input; x6k input; Pk input; z input
function [xkk,Pkk] = fcn(x1k,x2k,x3k,x4k,x5k,x6k,Pk,z)

% R = [2.782739102258347e-06 0 0 0 0 0;
%      0 1.936548166270313e-08 0 0 0 0;
%      0 0 2.718240466492716e-06 0 0 0;
%      0 0 0 1.809123162388460e-08 0 0;
%      0 0 0 0 5.587443411059212e-06 0;
%      0 0 0 0 0 5.587443411059212e-06];

R = [1.936548166270313e-08 0 0 0 0 0;
     0 2.782739102258347e-06 0 0 0 0;
     0 0 1.809123162388460e-08 0 0 0;
     0 0 0 2.718240466492716e-06 0 0;
     0 0 0 0 5.587443411059212e-06 0;
     0 0 0 0 0 2.976654513986432e-06];

H = [1 0 0 0 0 0;
     0 1 0 0 0 0;
     0 0 1 0 0 0;
     0 0 0 1 0 0;
     0 0 0 0 1 0;
     0 0 0 0 0 1];

xk = [x1k;x2k;x3k;x4k;x5k;x6k];

y = z - H * xk;

K = Pk*(H')/(H*Pk*(H') + R);

xkk = xk + K * y;
Pkk = (eye(6)-K * H) * Pk;

== matlab function PID_HW_EKF/EKF_quadcopter1/PROPAGATION ==
  data: x1 input; x1d output; x2 input; x3 input; x4 input; x5 input; x6 input; U_1 input; U_2 input; U_3 input; U_4 input; x2d output; x3d output; x4d output; x5d output; x6d output; Pk input; Pkp1 output
function [x1d,x2d,x3d,x4d,x5d,x6d,Pkp1] = fcn(x1,x2,x3,x4,x5,x6,U_1,U_2,U_3,U_4,Pk)

quadParams.g = 9.81;
quadParams.m = 1.07;
quadParams.Jx = 0.055;
quadParams.Jy = 0.055;
quadParams.Jz = 0.03;
quadParams.Jr=0;
quadParams.d = 0.1;
quadParams.L = 0.25;
quadParams.kd= 1.779e-07;  %Rotor torque coefficient(kg.m^2)   %M=kd*w^2
quadParams.kt = 1.105e-05;  %Rotor thrust coefficient(kg.m^2)  %T=kt*w^2

m = 1.07;
L = 0.25;
d = 0.055;
J = 0.055;
g = 9.81;
Ts = 0.002;

% Q = [0.0000000001 0 0 0 0 0;
%      0 0.00000001 0 0 0 0;
%      0 0 0.0000000001 0 0 0;
%      0 0 0 0.00000001 0 0;
%      0 0 0 0 0.0000000001 0;
%      0 0 0 0 0 0.00000001];

Q = [5e-16 0 0 0 0 0;
     0 1e-6 0 0 0 0;
     0 0 5e-16 0  0 0;
     0 0 0 1e-6 0 0;
     0 0 0 0 1e-13 0;
     0 0 0 0 0 5e-7];


a1=(quadParams.Jy-quadParams.Jz)/quadParams.Jx;
a2=-quadParams.Jr/quadParams.Jx;
a3=(quadParams.Jz-quadParams.Jx)/quadParams.Jy;
a4=quadParams.Jr/quadParams.Jy;
a5=(quadParams.Jx-quadParams.Jy)/quadParams.Jz;
b1=quadParams.L/quadParams.Jx;
b2=quadParams.L/quadParams.Jy;
b3=quadParams.L/quadParams.Jz;


x1d_dot =x2;

x2d_dot =x4*x6*a1 + b1*U_2;

x3d_dot =x4;

x4d_dot =x2*x6*a3+b2*U_3;

x5d_dot =x6;

x6d_dot =x4*x2*a5+b3*U_4;

x1d = x1 + x1d_dot*Ts;
x2d = x2 + x2d_dot*Ts;
x3d = x3 + x3d_dot*Ts;
x4d = x4 + x4d_dot*Ts;
x5d = x5 + x5d_dot*Ts;
x6d = x6 + x6d_dot*Ts;


F11 = 0;
F12 = 1;
F13 = 0;
F14 = 0;
F15 = 0;
F16 = 0;

F21 = 0;
F22 = 0;
F23 = 0;
F24 = x6*a1;
F25 = 0;
F26 = x4*a1;

F31 = 0;
F32 = 0;
F33 = 0;
F34 = 1;
F35 = 0;
F36 = 0;

F41 = 0;
F42 = x6*a3;
F43 = 0;
F44 = 0;
F45 = 0;
F46 = x2*a3;

F51 = 0;
F52 = 0;
F53 = 0;
F54 = 0;
F55 = 0;
F56 = 1;

F61 = 0;
F62 = x4*a5;
F63 = 0;
F64 = x2*a5;
F65 = 0;
F66 = 0;

F = [F11 F12 F13 F14 F15 F16;
     F21 F22 F23 F24 F25 F26;
     F31 F32 F33 F34 F35 F36;
     F41 F42 F43 F44 F45 F46;
     F51 F52 F53 F54 F55 F56;
     F61 F62 F63 F64 F65 F66];

PHI = expm(F * Ts);

Pkp1 = PHI * Pk * (PHI') + Q;
